simulink model "nonlinearAirframe"  (R2016b)
settings: Solver=ode3  StartTime=0  StopTime=10.0  FixedStep=Ts  RelTol=1e-3  EnableMultiTasking=on
undefined symbols (not defined in the file): Earth, initPosLLA, mass, thrustArm, Vehicle, WGS84
libraries: actuatorsLibrary x8, aerolib6dof2 x1, simulink x1, aerolibtransform2 x1
settings Model: Creator=The MathWorks, Inc.  LastModifiedBy=The MathWorks, Inc.
settings DataIOCC: LimitDataPoints=on  SaveFormat=Array  SaveOutput=off  SignalLogging=off  DSMLogging=off  SaveTime=off
settings OptimizationCC: BlockReduction=off  DefaultParameterBehavior=Inlined  BufferReuse=off  LifeSpan=inf
settings DebuggingCC: AlgebraicLoopMsg=none  UnderspecifiedInitializationDetection=Classic  MergeDetectMultiDrivingBlocksExec=none  UnconnectedInputMsg=none  UnconnectedOutputMsg=none  UnconnectedLineMsg=none  AllowSymbolicDim=off  SFUnexpectedBacktrackingDiag=warning  SFNoUnconditionalDefaultTransitionDiag=warning  SFExecutionAtInitializationDiag=none
settings HardwareCC: ProdBitPerPointer=32  ProdBitPerSizeT=32  ProdBitPerPtrDiffT=32  ProdLargestAtomicFloat=None  ProdIntDivRoundTo=Undefined  ProdEndianess=Unspecified  ProdWordSize=32  ProdHWDeviceType=32-bit Generic
settings ModelReferenceCC: PropagateSignalLabelsOutOfModel=off
settings GRTTargetCC: TargetLangStandard=C89/C90 (ANSI)  GeneratePreprocessorConditionals=Disable all
settings ConfigComp: CovMetricSettings=dw  CovHtmlReporting=on  CovSaveCumulativeToWorkspaceVar=on  CovSaveSingleToWorkspaceVar=on  CovExternalEMLEnable=off  CovSFcnEnable=off

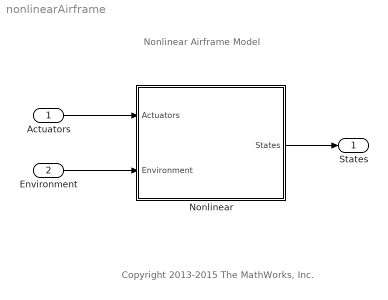
== system nonlinearAirframe ==
  note: Copyright 2013-2015 The MathWorks, Inc.
  note: Nonlinear Airframe Model
  Actuators : Inport  PortDimensions=[1 4]
  Environment : Inport  Port=2  OutDataTypeStr=Bus: EnvironmentBus  BusOutputAsStruct=on
  Nonlinear : Subsystem  TreatAsAtomicUnit=on
      mask init:
      | vehicleNonlinearVars;
  States : Outport  OutDataTypeStr=Bus: StatesBus  BusOutputAsStruct=on
  wires:
  Actuators/1 -> Nonlinear/1(Actuators)
  Environment/1 -> Nonlinear/2(Environment)
  Nonlinear/1(States) -> States/1

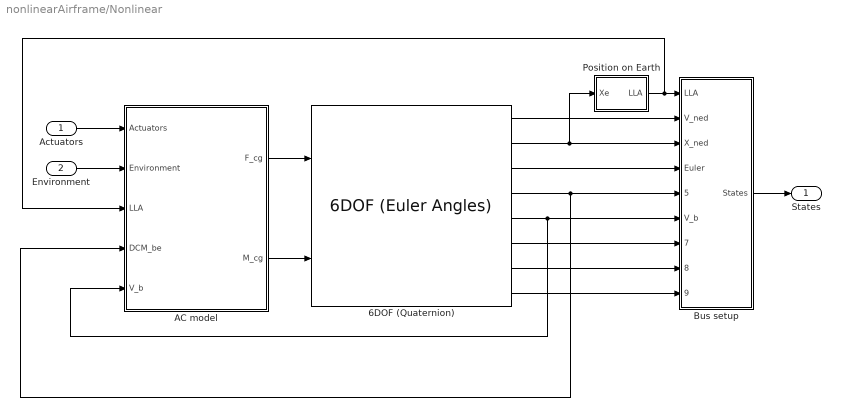
== system nonlinearAirframe/Nonlinear ==
  Actuators : Inport
  Environment : Inport  Port=2
  6DOF (Quaternion) : aerolib6dof2/6DOF (Euler Angles)  units=Metric (MKS)  mtype=Fixed  rep=Quaternion  xme_0=initPosNED  Vm_0=initVb  eul_0=initEuler  pm_0=initAngRates  mass_0=mass  mass_e=0.5  mass_f=2.0  inertia=inertia  inertia_e=eye(3)  inertia_f=2*eye(3)  k_quat=Vehicle.Nonlinear.Nonlinear.SixDOF.quatGain  vre_flag=on
  AC model : Subsystem
  Bus setup : Subsystem
  Position on Earth : Subsystem  Priority=1  TreatAsAtomicUnit=on
  States : Outport
  wires:
  Actuators/1 -> AC model/1(Actuators)
  Environment/1 -> AC model/2(Environment)
  AC model/1(F_cg) -> 6DOF (Quaternion)/1
  AC model/2(M_cg) -> 6DOF (Quaternion)/2
  6DOF (Quaternion)/1 -> Bus setup/2(V_ned)
  6DOF (Quaternion)/2 -> Bus setup/3(X_ned), Position on Earth/1(Xe)
  6DOF (Quaternion)/3 -> Bus setup/4(Euler)
  6DOF (Quaternion)/6 -> Bus setup/7(Omega_b)
  6DOF (Quaternion)/7 -> Bus setup/8(dOmega_b)
  6DOF (Quaternion)/8 -> Bus setup/9(Accel_b)
  Bus setup/1(States) -> States/1
  Position on Earth/1(LLA) -> AC model/3(LLA), Bus setup/1(LLA)
  6DOF (Quaternion)/5 -> AC model/5(V_b), Bus setup/6(V_b)
  6DOF (Quaternion)/4 -> AC model/4(DCM_be), Bus setup/5(DCM_be)

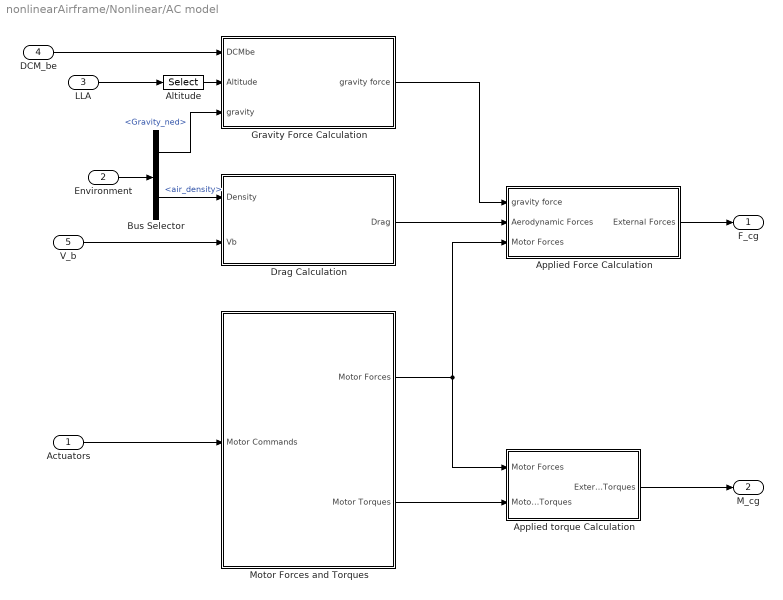
== system nonlinearAirframe/Nonlinear/AC model ==
  Actuators : Inport
  Environment : Inport  Port=2
  LLA : Inport  Port=3
  DCM_be : Inport  Port=4
  V_b : Inport  Port=5  Unit=m/s
  Altitude : Selector  InputPortWidth=3  IndexOptions=Index vector (dialog)  Indices=[3]  OutputSizes=1
  Applied Force Calculation : Subsystem
  Applied torque Calculation : Subsystem
  Bus Selector : BusSelector  OutputSignals=Gravity_ned,AtmosphereBus.air_density
  Drag Calculation : Subsystem
  Gravity Force Calculation : Subsystem
  Motor Forces and Torques : Subsystem
  F_cg : Outport  Unit=N
  M_cg : Outport  Port=2  Unit=N*m
  wires:
  Applied Force Calculation/1(External Forces) -> F_cg/1
  Applied torque Calculation/1(External Torques) -> M_cg/1
  Motor Forces and Torques/1(Motor Forces) -> Applied torque Calculation/1(Motor Forces), Applied Force Calculation/3(Motor Forces)
  Motor Forces and Torques/2(Motor Torques) -> Applied torque Calculation/2(Motor Torques)
  Bus Selector/1 -> Gravity Force Calculation/3(gravity)  "<Gravity_ned>"
  Gravity Force Calculation/1(gravity force) -> Applied Force Calculation/1(gravity force)
  Environment/1 -> Bus Selector/1
  Altitude/1 -> Gravity Force Calculation/2(Altitude)
  Bus Selector/2 -> Drag Calculation/1(Density)  "<air_density>"
  DCM_be/1 -> Gravity Force Calculation/1(DCMbe)
  LLA/1 -> Altitude/1
  V_b/1 -> Drag Calculation/2(Vb)
  Drag Calculation/1(Drag) -> Applied Force Calculation/2(Aerodynamic Forces)
  Actuators/1 -> Motor Forces and Torques/1(Motor Commands)

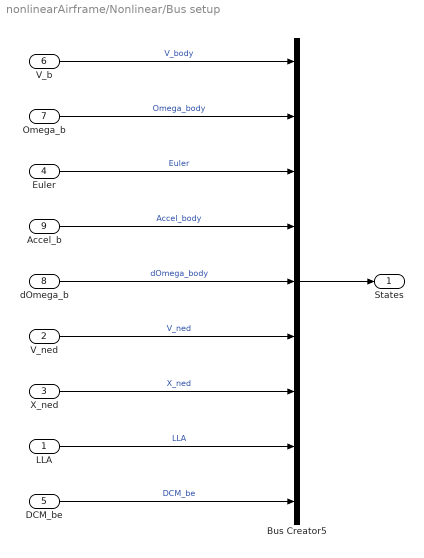
== system nonlinearAirframe/Nonlinear/Bus setup ==
  LLA : Inport  PortDimensions=3
  V_ned : Inport  Port=2  Unit=m/second  PortDimensions=3
  X_ned : Inport  Port=3  Unit=m  PortDimensions=3
  Euler : Inport  Port=4  Unit=rad  PortDimensions=3
  DCM_be : Inport  Port=5  PortDimensions=[3 3]
  V_b : Inport  Port=6  Unit=m/s  PortDimensions=3
  Omega_b : Inport  Port=7  Unit=rad/s  PortDimensions=3
  dOmega_b : Inport  Port=8  Unit=rad/s^2  PortDimensions=3
  Accel_b : Inport  Port=9  Unit=m/s^2  PortDimensions=3
  Bus Creator5 : BusCreator  Inputs=9  OutDataTypeStr=Bus: StatesBus  NonVirtualBus=on
  States : Outport
  wires:
  Bus Creator5/1 -> States/1
  V_b/1 -> Bus Creator5/1  "V_body"
  Omega_b/1 -> Bus Creator5/2  "Omega_body"
  Euler/1 -> Bus Creator5/3  "Euler"
  X_ned/1 -> Bus Creator5/7  "X_ned"
  Accel_b/1 -> Bus Creator5/4  "Accel_body"
  LLA/1 -> Bus Creator5/8  "LLA"
  dOmega_b/1 -> Bus Creator5/5  "dOmega_body"
  DCM_be/1 -> Bus Creator5/9  "DCM_be"
  V_ned/1 -> Bus Creator5/6  "V_ned"

== system nonlinearAirframe/Nonlinear/Position on Earth ==
  Xe : Inport  Unit=m
  Flat Earth to LLA : aerolibtransform2/Flat Earth to LLA  units=Metric (MKS)  ptype=Earth (WGS84)  F=1/298.257223563  R=6378137  LL0=initPosLLA(1:2)  psi=Vehicle.Nonlinear.Nonlinear.PositionOnEarth.FlatEarthToLLA.xAxis
  Mux : Mux  Inputs=2
  href : Constant  Value=Vehicle.Nonlinear.Nonlinear.PositionOnEarth.href
  LLA : Outport
  wires:
  Mux/1 -> LLA/1
  Xe/1 -> Flat Earth to LLA/1
  Flat Earth to LLA/1 -> Mux/1
  Flat Earth to LLA/2 -> Mux/2
  href/1 -> Flat Earth to LLA/2

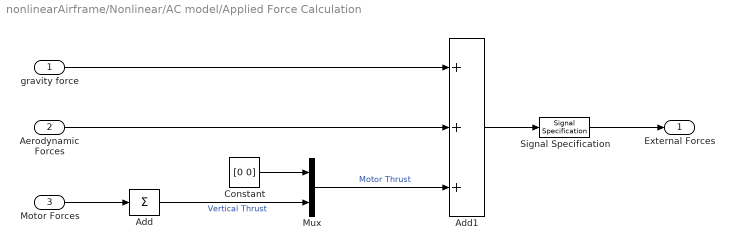
== system nonlinearAirframe/Nonlinear/AC model/Applied Force Calculation ==
  gravity force : Inport  Unit=N
  Aerodynamic Forces : Inport  Port=2  Unit=N
  Motor Forces : Inport  Port=3  Unit=N
  Add : Sum  Inputs=+
  Add1 : Sum  Inputs=+++
  Constant : Constant  Value=[0 0]
  Mux : Mux  Inputs=2
  Signal Specification : SignalSpecification  Dimensions=3
  External Forces : Outport  Unit=N
  wires:
  Add/1 -> Mux/2  "Vertical Thrust"
  Constant/1 -> Mux/1
  Add1/1 -> Signal Specification/1
  Motor Forces/1 -> Add/1
  Mux/1 -> Add1/3  "Motor Thrust"
  Aerodynamic Forces/1 -> Add1/2
  gravity force/1 -> Add1/1
  Signal Specification/1 -> External Forces/1

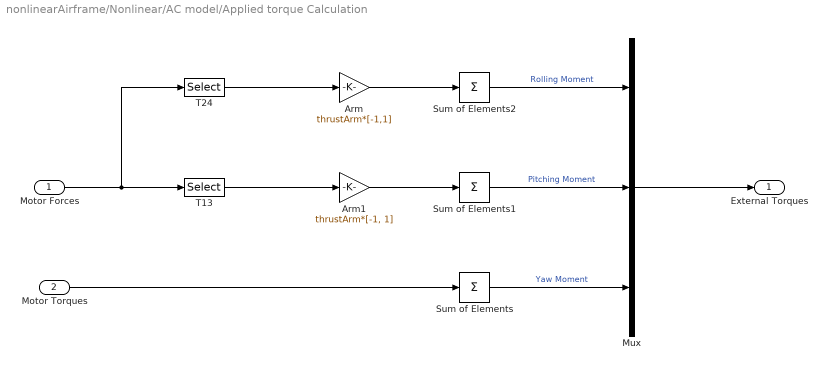
== system nonlinearAirframe/Nonlinear/AC model/Applied torque Calculation ==
  Motor Forces : Inport  Unit=N
  Motor Torques : Inport  Port=2  Unit=N*m
  Arm : Gain  Gain=thrustArm*[-1,1]
  Arm1 : Gain  Gain=thrustArm*[-1, 1]
  Mux : Mux  Inputs=3
  Sum of Elements : Sum  Inputs=+
  Sum of Elements1 : Sum  Inputs=+
  Sum of Elements2 : Sum  Inputs=+
  T13 : Selector  InputPortWidth=4  IndexOptions=Index vector (dialog)  Indices=[1 3]  OutputSizes=1
  T24 : Selector  InputPortWidth=4  IndexOptions=Index vector (dialog)  Indices=[2 4]  OutputSizes=1
  External Torques : Outport  Unit=N*m
  wires:
  Motor Torques/1 -> Sum of Elements/1
  Sum of Elements/1 -> Mux/3  "Yaw Moment"
  Motor Forces/1 -> T24/1, T13/1
  T13/1 -> Arm1/1
  T24/1 -> Arm/1
  Arm1/1 -> Sum of Elements1/1
  Sum of Elements1/1 -> Mux/2  "Pitching Moment"
  Arm/1 -> Sum of Elements2/1
  Sum of Elements2/1 -> Mux/1  "Rolling Moment"
  Mux/1 -> External Torques/1

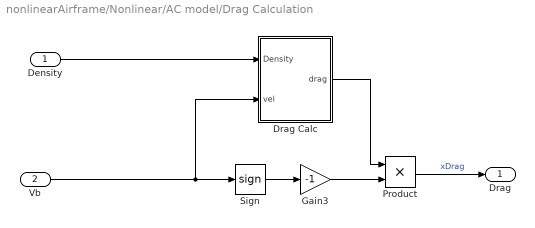
== system nonlinearAirframe/Nonlinear/AC model/Drag Calculation ==
  Density : Inport  Unit=kg/m^3
  Vb : Inport  Port=2  Unit=m/second
  Drag Calc : Subsystem
  Gain3 : Gain  Gain=-1
  Product : Product  RndMeth=Zero
  Sign : Signum  ZeroCross=off
  Drag : Outport  Unit=N
  wires:
  Density/1 -> Drag Calc/1(Density)
  Sign/1 -> Gain3/1
  Drag Calc/1(drag) -> Product/1
  Gain3/1 -> Product/2
  Product/1 -> Drag/1  "xDrag"
  Vb/1 -> Drag Calc/2(vel), Sign/1

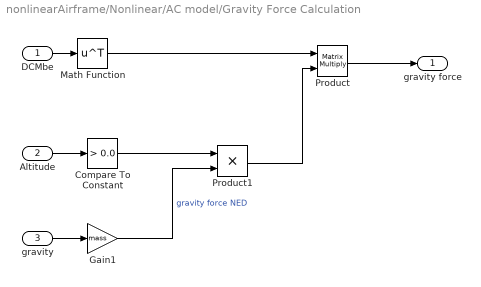
== system nonlinearAirframe/Nonlinear/AC model/Gravity Force Calculation ==
  DCMbe : Inport
  Altitude : Inport  Port=2  Unit=m
  gravity : Inport  Port=3  Unit=m/s^2
  Compare To Constant : simulink/Logic and Bit Operations/Compare To Constant  relop=>  const=0.0  OutDataTypeStr=boolean
  Gain1 : Gain  Gain=mass
  Math Function : Math  Operator=transpose  SaturateOnIntegerOverflow=on
  Product : Product  Multiplication=Matrix(*)
  Product1 : Product
  gravity force : Outport  Unit=N
  wires:
  gravity/1 -> Gain1/1
  Gain1/1 -> Product1/2  "gravity force NED"
  Product/1 -> gravity force/1
  Compare To Constant/1 -> Product1/1
  Product1/1 -> Product/2
  Altitude/1 -> Compare To Constant/1
  DCMbe/1 -> Math Function/1
  Math Function/1 -> Product/1

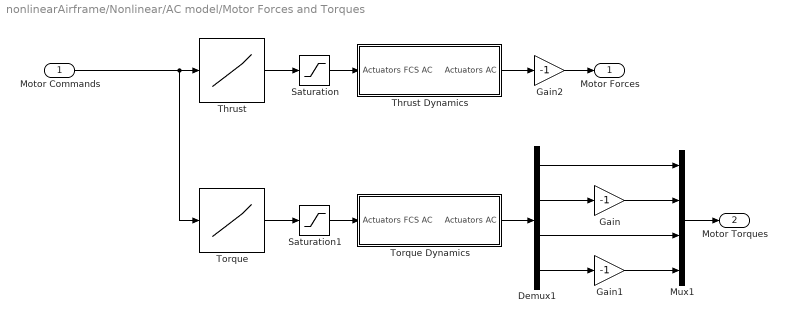
== system nonlinearAirframe/Nonlinear/AC model/Motor Forces and Torques ==
  Motor Commands : Inport
  Demux1 : Demux
  Gain : Gain  Gain=-1
  Gain1 : Gain  Gain=-1
  Gain2 : Gain  Gain=-1
  Mux1 : Mux
  Saturation : Saturate  UpperLimit=Vehicle.Nonlinear.Nonlinear.ACModel.ForcesMoments.Thrust.upperSat  LowerLimit=Vehicle.Nonlinear.Nonlinear.ACModel.ForcesMoments.Thrust.lowerSat
  Saturation1 : Saturate  UpperLimit=Vehicle.Nonlinear.Nonlinear.ACModel.ForcesMoments.Torque.upperSat  LowerLimit=Vehicle.Nonlinear.Nonlinear.ACModel.ForcesMoments.Torque.lowerSat
  Thrust : Lookup_n-D  NumberOfTableDimensions=1  BreakpointsForDimension1=Vehicle.Nonlinear.Nonlinear.ACModel.ForcesMoments.Thrust.breakpoints  Table=Vehicle.Nonlinear.Nonlinear.ACModel.ForcesMoments.Thrust.tableData  ExtrapMethod=Clip  UseLastTableValue=on  RndMeth=Simplest  InputSameDT=on
  Thrust Dynamics : Subsystem  Variant=on
  Torque : Lookup_n-D  NumberOfTableDimensions=1  BreakpointsForDimension1=Vehicle.Nonlinear.Nonlinear.ACModel.ForcesMoments.Torque.breakpoints  Table=Vehicle.Nonlinear.Nonlinear.ACModel.ForcesMoments.Torque.tableData  ExtrapMethod=Clip  UseLastTableValue=on  RndMeth=Simplest  InputSameDT=on
  Torque Dynamics : Subsystem  Variant=on
  Motor Forces : Outport  Unit=N
  Motor Torques : Outport  Port=2  Unit=N*m
  wires:
  Gain/1 -> Mux1/2
  Gain2/1 -> Motor Forces/1
  Torque Dynamics/1(Actuators AC) -> Demux1/1
  Thrust Dynamics/1(Actuators AC) -> Gain2/1
  Motor Commands/1 -> Torque/1, Thrust/1
  Mux1/1 -> Motor Torques/1
  Thrust/1 -> Saturation/1
  Torque/1 -> Saturation1/1
  Demux1/4 -> Gain1/1
  Saturation/1 -> Thrust Dynamics/1(Actuators FCS AC)
  Demux1/3 -> Mux1/3
  Demux1/2 -> Gain/1
  Saturation1/1 -> Torque Dynamics/1(Actuators FCS AC)
  Demux1/1 -> Mux1/1
  Gain1/1 -> Mux1/4

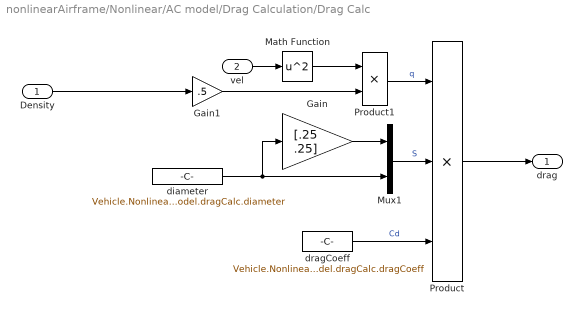
== system nonlinearAirframe/Nonlinear/AC model/Drag Calculation/Drag Calc ==
  Density : Inport  Unit=kg/m^3
  vel : Inport  Port=2  Unit=m/s
  Gain : Gain  Gain=[.25 .25]
  Gain1 : Gain  Gain=.5
  Math Function : Math  Operator=square  SaturateOnIntegerOverflow=on
  Mux1 : Mux  Inputs=2
  Product : Product  Inputs=3  RndMeth=Zero
  Product1 : Product  RndMeth=Zero
  diameter : Constant  Value=Vehicle.Nonlinear.Nonlinear.ACModel.dragCalc.diameter  SampleTime=0
  dragCoeff : Constant  Value=Vehicle.Nonlinear.Nonlinear.ACModel.dragCalc.dragCoeff  SampleTime=0
  drag : Outport  Unit=N
  wires:
  Product/1 -> drag/1
  dragCoeff/1 -> Product/3  "Cd"
  vel/1 -> Math Function/1
  Product1/1 -> Product/1  "q"
  diameter/1 -> Gain/1, Mux1/2
  Mux1/1 -> Product/2  "S"
  Gain/1 -> Mux1/1
  Gain1/1 -> Product1/2
  Math Function/1 -> Product1/1
  Density/1 -> Gain1/1

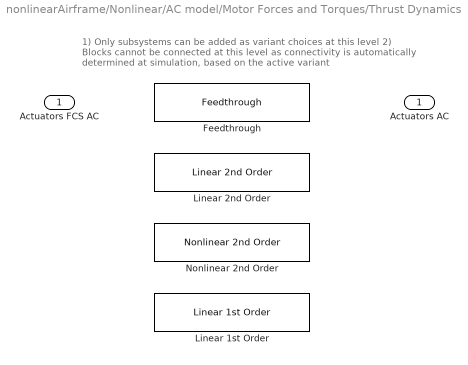
== system nonlinearAirframe/Nonlinear/AC model/Motor Forces and Torques/Thrust Dynamics ==
  note: 1) Only subsystems can be added as variant choices at this level
      | 2) Blocks cannot be connected at this level as connectivity is
      | automatically determined at simulation, based on the active variant
  Actuators FCS AC : Inport
  Feedthrough : actuatorsLibrary/Feedthrough  VariantControl=Variants.Actuators == 0
  Linear 1st Order : actuatorsLibrary/Linear 1st Order  VariantControl=Variants.Actuators == 3  a=Vehicle.Nonlinear.Nonlinear.ACModel.Actuator.LinearFirst.invTs
  Linear 2nd Order : actuatorsLibrary/Linear 2nd Order  VariantControl=Variants.Actuators == 1
  Nonlinear 2nd Order : actuatorsLibrary/Nonlinear 2nd Order  VariantControl=Variants.Actuators == 2
  Actuators AC : Outport

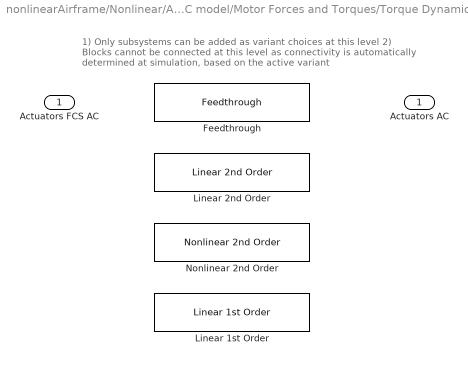
== system nonlinearAirframe/Nonlinear/AC model/Motor Forces and Torques/Torque Dynamics ==
  note: 1) Only subsystems can be added as variant choices at this level
      | 2) Blocks cannot be connected at this level as connectivity is
      | automatically determined at simulation, based on the active variant
  Actuators FCS AC : Inport
  Feedthrough : actuatorsLibrary/Feedthrough  VariantControl=Variants.Actuators == 0
  Linear 1st Order : actuatorsLibrary/Linear 1st Order  VariantControl=Variants.Actuators == 3  a=Vehicle.Nonlinear.Nonlinear.ACModel.Actuator.LinearFirst.invTs
  Linear 2nd Order : actuatorsLibrary/Linear 2nd Order  VariantControl=Variants.Actuators == 1
  Nonlinear 2nd Order : actuatorsLibrary/Nonlinear 2nd Order  VariantControl=Variants.Actuators == 2
  Actuators AC : Outport
